simulink model "Temparature_Control_Using_FlowChart"  (R2025b)
settings: Solver=FixedStepDiscrete  StartTime=0.0  StopTime=10.0  FixedStep=0.01  RelTol=1e-3
libraries: simulink x2
settings Model: Creator=soura  LastModifiedBy=soura

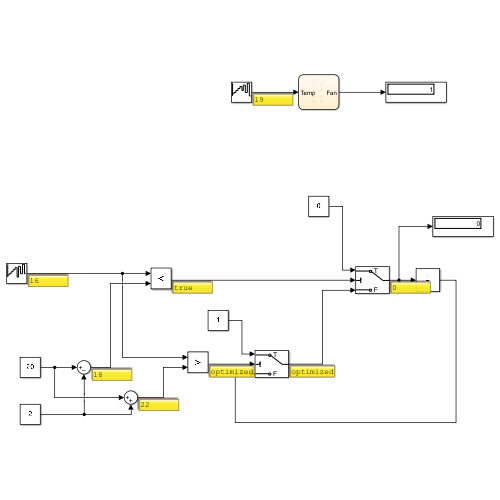
[thumbnail: Simulink's stored preview of the top-level diagram]
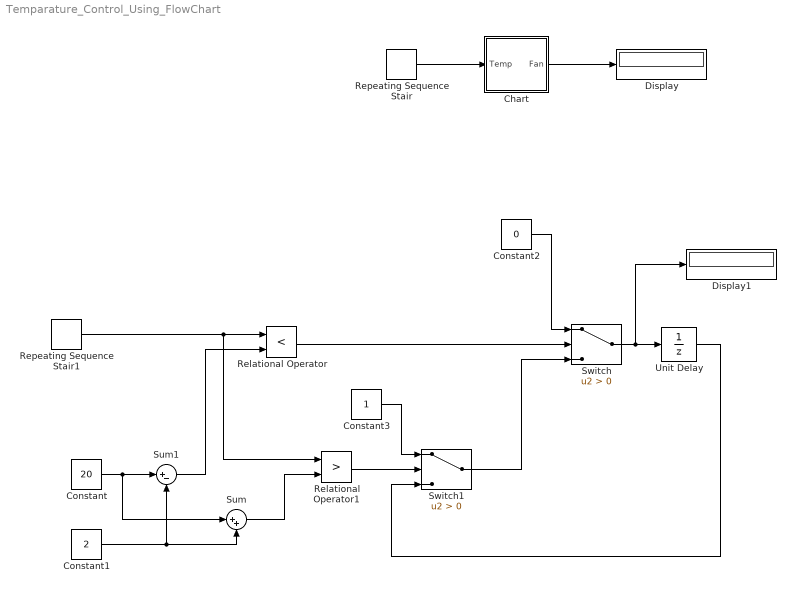
== system Temparature_Control_Using_FlowChart ==
  Chart : Stateflow chart  TreatAsAtomicUnit=on
  Constant : Constant  Value=20
  Constant1 : Constant  Value=2
  Constant2 : Constant  Value=0
  Constant3 : Constant
  Display : Display
  Display1 : Display
  Relational Operator : RelationalOperator  Operator=<  OutDataTypeStr=boolean  RndMeth=Simplest  InputSameDT=off
  Relational Operator1 : RelationalOperator  Operator=>  OutDataTypeStr=boolean  RndMeth=Simplest  InputSameDT=off
  Repeating Sequence Stair : simulink/Sources/Repeating Sequence Stair  OutValues=[17 18 19 20 21 19 22 18 23 16].'  tsamp=-1  OutMin=[]  OutMax=[]  OutDataTypeStr=double  OutputDataTypeScalingMode=double  OutDataType=fixdt(0,8)  ConRadixGroup=Best Precision: Vector-wise  OutScaling=2^-12
  Repeating Sequence Stair1 : simulink/Sources/Repeating Sequence Stair  OutValues=[17 18 19 20 21 16 22 18 23 18].'  tsamp=-1  OutMin=[]  OutMax=[]  OutDataTypeStr=double  OutputDataTypeScalingMode=double  OutDataType=fixdt(0,8)  ConRadixGroup=Best Precision: Vector-wise  OutScaling=2^-12
  Sum : Sum  Inputs=|++
  Sum1 : Sum  Inputs=|+-
  Switch : Switch  Criteria=u2 > Threshold  SaturateOnIntegerOverflow=off  InputSameDT=off
  Switch1 : Switch  Criteria=u2 > Threshold  SaturateOnIntegerOverflow=off  InputSameDT=off
  Unit Delay : UnitDelay  SampleTime=-1  HasFrameUpgradeWarning=on
  wires:
  Repeating Sequence Stair/1 -> Chart/1(Temp)
  Chart/1(Fan) -> Display/1
  Constant/1 -> Sum/1, Sum1/1
  Constant1/1 -> Sum/2, Sum1/2
  Repeating Sequence Stair1/1 -> Relational Operator1/1, Relational Operator/1
  Sum1/1 -> Relational Operator/2
  Relational Operator/1 -> Switch/2
  Constant2/1 -> Switch/1
  Sum/1 -> Relational Operator1/2
  Relational Operator1/1 -> Switch1/2
  Constant3/1 -> Switch1/1
  Switch1/1 -> Switch/3
  Switch/1 -> Display1/1, Unit Delay/1
  Unit Delay/1 -> Switch1/3

== stateflow chart Temparature_Control_Using_FlowChart/Chart ==
  (default) -> (junction 1)
  (junction 1) -> (junction 2)
  (junction 2) -> (junction 5) [order 1] : [Temp>20]
  (junction 2) -> (junction 7) [order 2]
  (junction 5) -> (junction 9) : {Fan=1;}
  (junction 9) -> (junction 7)
  (junction 7) -> (junction 11)
  (junction 11) -> (junction 14) [order 1] : [Temp<18]
  (junction 11) -> (junction 16) [order 2]
  (junction 14) -> (junction 18) : {Fan=0;}
  (junction 18) -> (junction 16)
  (junction 16) -> (junction 21)
  data: Temp input; Fan output
